simulink model "MBK_ControlSystem"  (R2025a)
settings: Solver=VariableStepAuto  StartTime=0.0  StopTime=10.0  RelTol=1e-3
values from neighbouring files (symbols this model uses):
  CF = 100    [MBK_param.m]
  Ga = 14    [MBK_param.m]
  Gp = Ye*Ym*n*Kt/(1+n^2*Kb*Kt*Ye*Ym)*1/s    [MBK_param.m]
  N = 0.5+Nf    [MBK_param.m]
undefined symbols (not defined in the file or in its folder): Nd
settings Model: Creator=ethan  LastModifiedBy=ethan

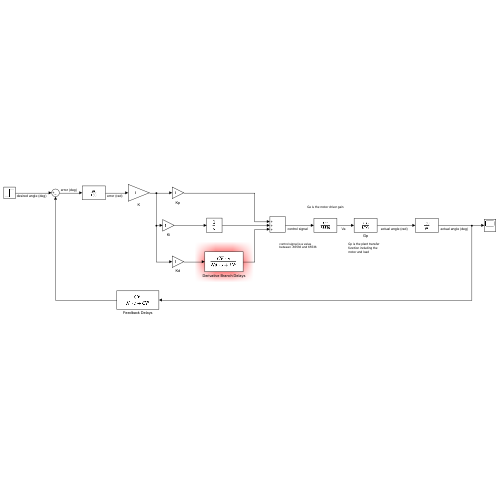
[thumbnail: Simulink's stored preview of the top-level diagram]
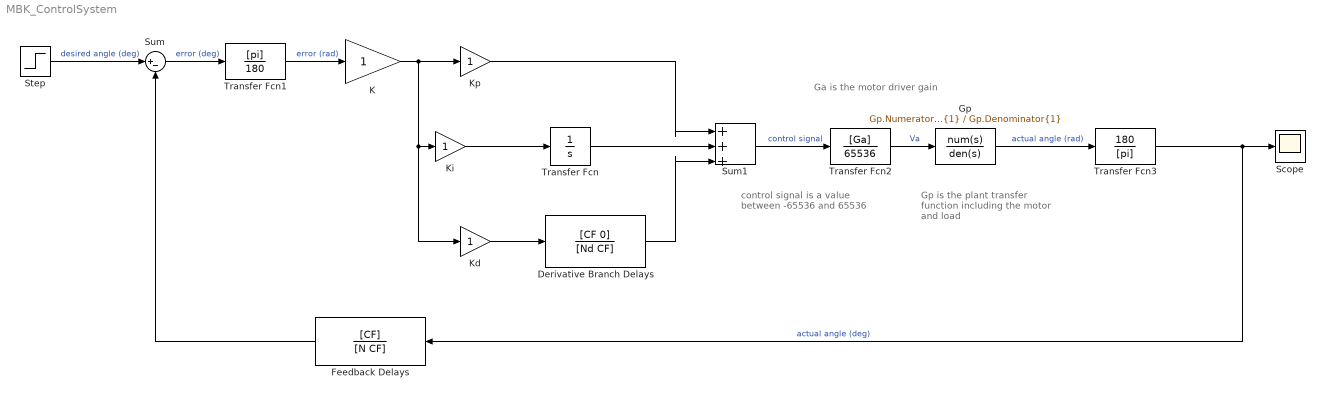
== system MBK_ControlSystem ==
  note: Gp is the plant transfer function including the motor and load
  note: Ga is the motor driver gain
  note: control signal is a value between -65536 and 65536
  Derivative Branch Delays : TransferFcn  Numerator=[CF 0]  Denominator=[Nd CF]
  Feedback Delays : TransferFcn  Numerator=[CF]  Denominator=[N CF]
  Gp : TransferFcn  Numerator=Gp.Numerator{1}  Denominator=Gp.Denominator{1}
  K : Gain
  Kd : Gain
  Ki : Gain
  Kp : Gain
  Scope : Scope
  Step : Step  SampleTime=0
  Sum : Sum  Inputs=|+-
  Sum1 : Sum  Inputs=|+|+|+
  Transfer Fcn : TransferFcn  Denominator=[1 0]
  Transfer Fcn1 : TransferFcn  Numerator=[pi]  Denominator=[180]
  Transfer Fcn2 : TransferFcn  Numerator=[Ga]  Denominator=[65536]
  Transfer Fcn3 : TransferFcn  Numerator=[180]  Denominator=[pi]
  wires:
  K/1 -> Kd/1, Ki/1, Kp/1
  Kd/1 -> Derivative Branch Delays/1
  Ki/1 -> Transfer Fcn/1
  Derivative Branch Delays/1 -> Sum1/3
  Transfer Fcn/1 -> Sum1/2
  Kp/1 -> Sum1/1
  Sum/1 -> Transfer Fcn1/1  "error (deg)"
  Step/1 -> Sum/1  "desired angle (deg)"
  Feedback Delays/1 -> Sum/2
  Sum1/1 -> Transfer Fcn2/1  "control signal"
  Transfer Fcn2/1 -> Gp/1  "Va"
  Transfer Fcn1/1 -> K/1  "error (rad)"
  Gp/1 -> Transfer Fcn3/1  "actual angle (rad)"
  Transfer Fcn3/1 -> Feedback Delays/1, Scope/1  "actual angle (deg)"
